simulink library "sf_bidder"  (Simulink 6.0)
settings: Solver=ode45  SolverMode=SingleTasking  StartTime=0.0  StopTime=10.0  RelTol=1e-3
settings Model: CovMetricSettings=dcmtr  Creator=The MathWorks Inc.  LastModifiedBy=batserve  ExtModeAutoUpdateStatusClock=off
settings OptimizationCC: BooleanDataType=off
settings DebuggingCC: CheckExecutionContextPreStartOutputMsg=on  CheckExecutionContextRuntimeOutputMsg=on  SolverPrmCheckMsg=none
settings HardwareCC: TargetUnknown=on

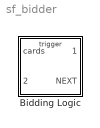
== system sf_bidder ==
  Bidding Logic : Stateflow chart  PropExecContextAcrossSSBoundary=on

== stateflow chart Bidding Logic ==
  state bid() [function]
    (default) -> (junction 18)
    (junction 18) -> (junction 19) : {
        | $ $
        | /* Condition 1: Open 1N */
        | c1 = (point_count>=16&&point_count<=18);
        | }
    (junction 19) -> (junction 20) : {
        | $ $
        | /* Condition 2: Open 2N */
        | c2 = (point_count>=20);
        | }
    (junction 20) -> (junction 21) : {
        | $ $
        | /* Condition 3: Open 2C */
        | c3 = (total_points>=22);
        | }
    (junction 21) -> (junction 22) : {
        | $ $
        | /* Condition 4: Opening Count */
        | c4 = (total_points>=13);
        | }
    (junction 22) -> (junction 23) : {
        | $ $
        | /* Condition 5: Premptable Count */
        | c5 = (point_count>=6);
        | }
    (junction 23) -> (junction 24) : {
        | $ $
        | /* Condition 6: Bid Spades */
        | c6 = (spade_count >= 5);
        | }
    (junction 24) -> (junction 25) : {
        | $ $
        | /* Condition 7: Bid Hearts */
        | c7 = (heart_count >= 5);
        | }
    (junction 25) -> (junction 26) : {
        | $ $
        | /* Condition 8: Bid Diamonds */
        | c8 = (diamond_count >= 4);
        | }
    (junction 26) -> (junction 27) : {
        | $ $
        | /* Condition 9: Preempt Spades */
        | c9 = (spade_count >=6);
        | }
    (junction 27) -> (junction 28) : {
        | $ $
        | /* Condition 10: Preempt Hearts */
        | c10 = (heart_count >=6);
        | }
    (junction 28) -> (junction 29) : {
        | $ $
        | /* Condition 11: Preempt Diamonds */
        | c11 = (diamond_count >= 6);
        | }
    (junction 29) -> (junction 30) : {
        | $ $
        | /* Condition 12: Even Distribution */
        | c12 = (distribution_count <= 1);
        | }
    (junction 30) -> (junction 31) : [c3&&!c12]   /* D1 */
    (junction 31) -> (junction 32) : {
        | $ $
        | /* Action 2: Bid 2 */
        | bid_out += 2;
        | }
    (junction 32) -> (junction 33) : {
        | $ $
        | /* Action 'CLUBS': Bid Clubs */
        | bid_out += club_mask;
        | }
    (junction 30) -> (junction 34)
    (junction 34) -> (junction 35) : [c2&&c12]   /* D2 */
    (junction 35) -> (junction 36) : {
        | $ $
        | /* Action 2: Bid 2 */
        | bid_out += 2;
        | }
    (junction 36) -> (junction 37) : {
        | $ $
        | /* Action 'NO_TRUMP': Bid No Trump */
        | bid_out += no_trump_mask;
        | }
    (junction 34) -> (junction 38)
    (junction 38) -> (junction 39) : [c1&&c12]   /* D3 */
    (junction 39) -> (junction 40) : {
        | $ $
        | /* Action 1: Bid 1 */
        | bid_out += 1;
        | }
    (junction 40) -> (junction 41) : {
        | $ $
        | /* Action 'NO_TRUMP': Bid No Trump */
        | bid_out += no_trump_mask;
        | }
    (junction 38) -> (junction 42)
    (junction 42) -> (junction 43) : [c4&&c6]   /* D4 */
    (junction 43) -> (junction 44) : {
        | $ $
        | /* Action 1: Bid 1 */
        | bid_out += 1;
        | }
    (junction 44) -> (junction 45) : {
        | $ $
        | /* Action 'SPADES': Bid Spades */
        | bid_out += spade_mask;
        | }
    (junction 42) -> (junction 46)
    (junction 46) -> (junction 47) : [c4&&c7]   /* D5 */
    (junction 47) -> (junction 48) : {
        | $ $
        | /* Action 1: Bid 1 */
        | bid_out += 1;
        | }
    (junction 48) -> (junction 49) : {
        | $ $
        | /* Action 'HEARTS': Bid Hearts */
        | bid_out += heart_mask;
        | }
    (junction 46) -> (junction 50)
    (junction 50) -> (junction 51) : [c4&&c8]   /* D6 */
    (junction 51) -> (junction 52) : {
        | $ $
        | /* Action 1: Bid 1 */
        | bid_out += 1;
        | }
    (junction 52) -> (junction 53) : {
        | $ $
        | /* Action 'DIAMONDS': Bid Diamonds */
        | bid_out += diamond_mask;
        | }
    (junction 50) -> (junction 54)
    (junction 54) -> (junction 55) : [c4]   /* D7 */
    (junction 55) -> (junction 56) : {
        | $ $
        | /* Action 1: Bid 1 */
        | bid_out += 1;
        | }
    (junction 56) -> (junction 57) : {
        | $ $
        | /* Action 'CLUBS': Bid Clubs */
        | bid_out += club_mask;
        | }
    (junction 54) -> (junction 58)
    (junction 58) -> (junction 59) : [c5&&c9]   /* D8 */
    (junction 59) -> (junction 60) : {
        | $ $
        | /* Action 2: Bid 2 */
        | bid_out += 2;
        | }
    (junction 60) -> (junction 61) : {
        | $ $
        | /* Action 'SPADES': Bid Spades */
        | bid_out += spade_mask;
        | }
    (junction 58) -> (junction 62)
    (junction 62) -> (junction 63) : [c5&&c10]   /* D9 */
    (junction 63) -> (junction 64) : {
        | $ $
        | /* Action 2: Bid 2 */
        | bid_out += 2;
        | }
    (junction 64) -> (junction 65) : {
        | $ $
        | /* Action 'HEARTS': Bid Hearts */
        | bid_out += heart_mask;
        | }
    (junction 62) -> (junction 66)
    (junction 66) -> (junction 67) : [c5&&c11]   /* D10 */
    (junction 67) -> (junction 68) : {
        | $ $
        | /* Action 2: Bid 2 */
        | bid_out += 2;
        | }
    (junction 68) -> (junction 69) : {
        | $ $
        | /* Action 'DIAMONDS': Bid Diamonds */
        | bid_out += diamond_mask;
        | }
    (junction 66) -> (junction 70)
    (junction 70) -> (junction 71) : /* Default */
    (junction 71) -> (junction 72) : {
        | $ $
        | /* Action 'PASS': Pass */
        | bid_out = 0;
        | }
  state points = count_distribution(suit_count) [function]
    (junction 7) -> (junction 8) : [suit_count < 3] {points = 3-suit_count;}
    (junction 7) -> (junction 6) : {points = 0;}
    (default) -> (junction 7)
  (default) -> (junction 5) : DEAL
      | {
      | loop = 0;
      | point_count = 0;
      | distribution_count = 0;
      | club_count = 0;
      | diamond_count = 0;
      | heart_count = 0;
      | spade_count = 0;
      | }
  (junction 5) -> (junction 11) : [loop<13]
      | {
      | club_count += (cards[loop]&club_mask)>0;
      | diamond_count += (cards[loop]&diamond_mask)>0;
      | heart_count += (cards[loop]&heart_mask)>0;
      | spade_count += (cards[loop]&spade_mask)>0;
      | }
  (junction 5) -> (junction 9)
  (default) -> (junction 10) : BID
      | {bid_out = 0;}
  (junction 9) -> (junction 17) : {
      | distribution_count += count_distribution(club_count);
      | distribution_count += count_distribution(diamond_count);
      | distribution_count += count_distribution(heart_count);
      | distribution_count += count_distribution(spade_count);
      | total_points = distribution_count+point_count;
      | }
  (junction 13) -> (junction 5) : {loop++;}
  (junction 12) -> (junction 13)
  (junction 14) -> (junction 12)
  (junction 11) -> (junction 14) : [cards[loop] & honor_mask]
      | {point_count+=cards[loop]&card_mask;}
  (junction 11) -> (junction 13)
  (junction 10) -> (junction 16) : {NEXT;}
  (junction 10) -> (junction 15) : [bid_in == 0]
      | {bid();NEXT;}
  data: c1 temporary boolean size=1; c2 temporary boolean size=1; c3 temporary boolean size=1; c4 temporary boolean size=1; c5 temporary boolean size=1; c6 temporary boolean size=1; c7 temporary boolean size=1; c8 temporary boolean size=1; c9 temporary boolean size=1; c10 temporary boolean size=1; c11 temporary boolean size=1; c12 temporary boolean size=1; suit_count function_input double size=1; points function_output double size=1; club_mask constant uint8 size=1 =0x10; diamond_mask constant uint8 size=1 =0x20; heart_mask constant uint8 size=1 =0x40; spade_mask constant uint8 size=1 =0x80; honor_mask constant uint8 size=1 =0x08; point_count local uint8 size=1; club_count local uint8 size=1; diamond_count local uint8 size=1; heart_count local uint8 size=1; spade_count local uint8 size=1; distribution_count local uint8 size=1; total_points local uint8 size=1; loop local uint8 size=1; cards input uint8 size=13; card_mask constant uint8 size=1 =0x07; bid_in input uint8 size=1; bid_out output uint8 size=1; no_trump_mask constant uint8 size=1 =0x08; double_mask constant uint8 size=1 =0x10; redouble_mask constant uint8 size=1 =0x20
  data c1 settings: description=Open 1N
  data c2 settings: description=Open 2N
  data c3 settings: description=Open 2C
  data c4 settings: description=Opening Count
  data c5 settings: description=Premptable Count
  data c6 settings: description=Bid Spades
  data c7 settings: description=Bid Hearts
  data c8 settings: description=Bid Diamonds
  data c9 settings: description=Preempt Spades
  data c10 settings: description=Preempt Hearts
  data c11 settings: description=Preempt Diamonds
  data c12 settings: description=Even Distribution
  events: DEAL input EITHER_EDGE_EVENT; BID input EITHER_EDGE_EVENT; NEXT output EITHER_EDGE_EVENT
